simulink model "model2"  (R2013a)
settings: Solver=ode45  StartTime=0.0  StopTime=10.0  RelTol=1e-3
undefined symbols (not defined in the file): k77
settings Model: Creator=Axel  LastModifiedBy=Axel
settings OptimizationCC: InlineParams=on

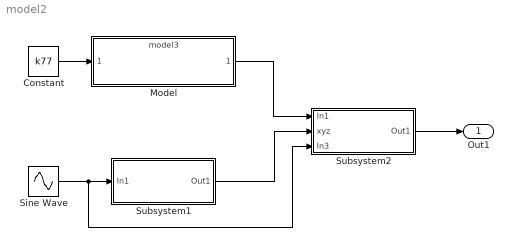
== system model2 ==
  Constant : Constant  Value=k77
  Model : ModelReference  ModelNameDialog=model3.slx  SimulationMode=Normal  ModelReferenceVersion=1.4  CopyOfModelName=model3.slx  DefaultDataLogging=on
  Sine Wave : Sin  SampleTime=0
  Subsystem1 : Subsystem
  Subsystem2 : Subsystem
  Out1 : Outport
  wires:
  Sine Wave/1 -> Subsystem2/3(In3), Subsystem1/1(In1)
  Subsystem1/1(Out1) -> Subsystem2/2(xyz)
  Subsystem2/1(Out1) -> Out1/1
  Constant/1 -> Model/1
  Model/1 -> Subsystem2/1(In1)

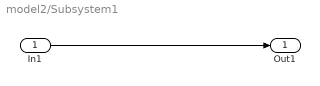
== system model2/Subsystem1 ==
  In1 : Inport
  Out1 : Outport
  wires:
  In1/1 -> Out1/1

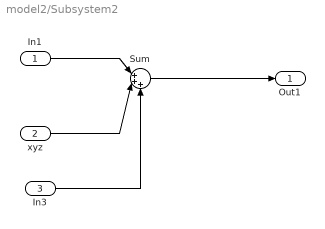
== system model2/Subsystem2 ==
  In1 : Inport
  xyz : Inport  Port=2
  In3 : Inport  Port=3
  Sum : Sum  Inputs=|+++
  Out1 : Outport
  wires:
  xyz/1 -> Sum/2
  In1/1 -> Sum/1
  Sum/1 -> Out1/1
  In3/1 -> Sum/3
